simulink model "RCN_comparation"  (R2014b)
settings: Solver=ode45  StartTime=0.0  StopTime=4  RelTol=1e-3
libraries: NeuroModelerLibrary x31, simulink x4
settings Model: Creator=ai?  LastModifiedBy=Tim
settings DataIOCC: SignalLoggingSaveFormat=ModelDataLogs
settings OptimizationCC: ExpressionDepthLimit=2147483647
settings DebuggingCC: UnderspecifiedInitializationDetection=Classic  MergeDetectMultiDrivingBlocksExec=none  FcnCallInpInsideContextMsg=UseLocalSettings  StateNameClashWarn=warning
settings GRTTargetCC: CombineOutputUpdateFcns=off  GRTInterface=on

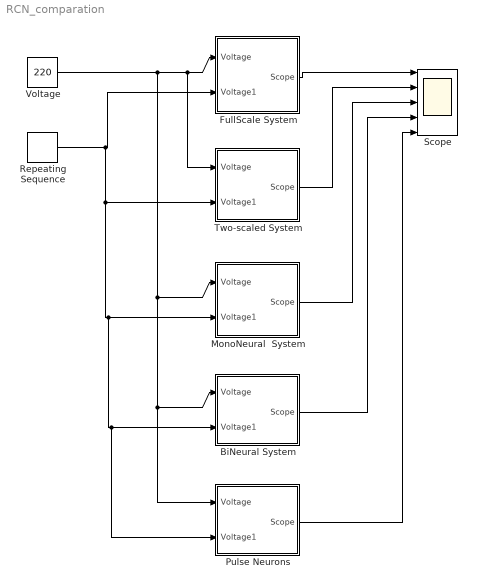
== system RCN_comparation ==
  BiNeural System : Subsystem
  FullScale System : Subsystem
  MonoNeural  System : Subsystem
  Pulse Neurons : Subsystem
  Repeating Sequence : simulink/Sources/Repeating Sequence  rep_seq_t=[0 1 1.01 2 2.01 3 3.01 4 4.01 10]  rep_seq_y=[3 3 1 1 -2 -2 -1 -1 20 20]
  Scope : Scope  NumInputPorts=5
      settings: YMin=0~0~0~0~-500  YMax=5~200~4~4~500  MaxDataPoints=500000
  Two-scaled System : Subsystem
  Voltage : Constant  Value=220
  wires:
  FullScale System/1(Scope) -> Scope/1
  Two-scaled System/1(Scope) -> Scope/2
  MonoNeural  System/1(Scope) -> Scope/3
  BiNeural System/1(Scope) -> Scope/4
  Pulse Neurons/1(Scope) -> Scope/5
  Voltage/1 -> FullScale System/1(Voltage), Two-scaled System/1(Voltage), MonoNeural  System/1(Voltage), BiNeural System/1(Voltage), Pulse Neurons/1(Voltage)
  Repeating Sequence/1 -> Pulse Neurons/2(Voltage1), BiNeural System/2(Voltage1), MonoNeural  System/2(Voltage1), Two-scaled System/2(Voltage1), FullScale System/2(Voltage1)

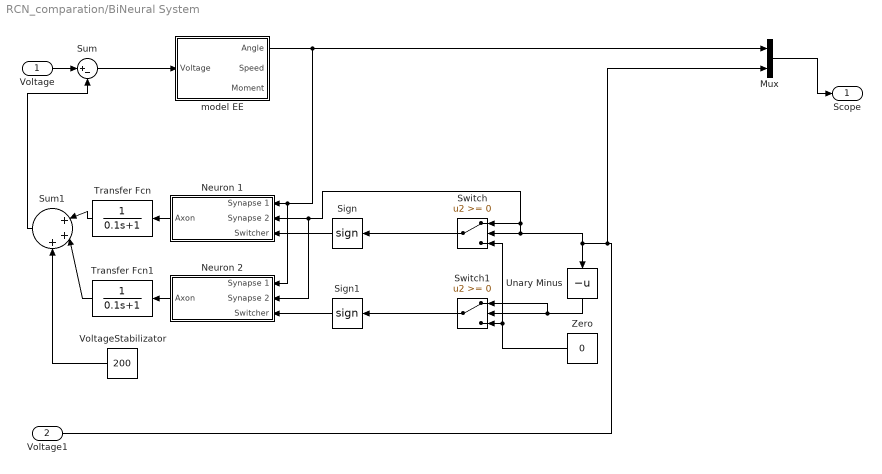
== system RCN_comparation/BiNeural System ==
  Voltage : Inport
  Voltage1 : Inport  Port=2
  Mux : Mux  Inputs=2
  Neuron 1 : Subsystem
  Neuron 2 : Subsystem
  Sign : Signum
  Sign1 : Signum
  Sum : Sum  Inputs=|+-
  Sum1 : Sum  Inputs=|+++
  Switch : Switch
  Switch1 : Switch
  Transfer Fcn : TransferFcn  Denominator=[0.1 1]
  Transfer Fcn1 : TransferFcn  Denominator=[0.1 1]
  Unary Minus : UnaryMinus
  VoltageStabilizator : Constant  Value=200
  Zero : Constant  Value=0
  model EE : Subsystem
  Scope : Outport
  wires:
  model EE/1(Angle) -> Mux/1, Neuron 1/1(Synapse 1), Neuron 2/1(Synapse 1)
  Voltage/1 -> Sum/1
  Mux/1 -> Scope/1
  Sum/1 -> model EE/1(Voltage)
  Neuron 1/1(Axon) -> Transfer Fcn/1
  Sum1/1 -> Sum/2
  Neuron 2/1(Axon) -> Transfer Fcn1/1
  Switch/1 -> Sign/1
  Switch1/1 -> Sign1/1
  Unary Minus/1 -> Switch1/2, Switch1/1
  Zero/1 -> Switch1/3, Switch/3
  Sign1/1 -> Neuron 2/3(Switcher)
  Sign/1 -> Neuron 1/3(Switcher)
  Transfer Fcn/1 -> Sum1/1
  Transfer Fcn1/1 -> Sum1/2
  VoltageStabilizator/1 -> Sum1/3
  Voltage1/1 -> Mux/2, Unary Minus/1, Neuron 2/2(Synapse 2), Neuron 1/2(Synapse 2), Switch/1, Switch/2

== system RCN_comparation/FullScale System ==
  Voltage : Inport
  Voltage1 : Inport  Port=2
  Angle Needed : Constant  Value=3
  Control Unit : Subsystem
  Manual Switch : ManualSwitch  CurrentSetting=0
  Mux : Mux  Inputs=2
  PID Controller : simulink/Continuous/PID Controller  Controller=PI  TimeDomain=Continuous-time  SampleTime=-1  IntegratorMethod=Forward Euler  FilterMethod=Forward Euler  Form=Parallel  P=1.41465294803961  I=22.6639520121412  D=0.242701786704104  N=12.4632340746272  InitialConditionSource=internal  InitialConditionForIntegrator=0  InitialConditionForFilter=0  ExternalReset=none  LimitOutput=off  UpperSaturationLimit=inf  LowerSaturationLimit=-inf  LinearizeAsGain=off  AntiWindupMode=none  Kb=1  TrackingMode=off  Kt=1  PParamMin=[]  PParamMax=[]  IParamMin=[]  IParamMax=[]  DParamMin=[]  DParamMax=[]  NParamMin=[]  NParamMax=[]  KbParamMin=[]  KbParamMax=[]  KtParamMin=[]  KtParamMax=[]  POutMin=[]  POutMax=[]  IOutMin=[]  IOutMax=[]  DOutMin=[]  DOutMax=[]  NOutMin=[]  NOutMax=[]  KbOutMin=[]  KbOutMax=[]  KtOutMin=[]  KtOutMax=[]  IntegratorOutMin=[]  IntegratorOutMax=[]  FilterOutMin=[]  FilterOutMax=[]  SumOutMin=[]  SumOutMax=[]  SumI1OutMin=[]  SumI1OutMax=[]  SumI2OutMin=[]  SumI2OutMax=[]  SumI3OutMin=[]  SumI3OutMax=[]  SumDOutMin=[]  SumDOutMax=[]  SaturationOutMin=[]  SaturationOutMax=[]  IntegratorContinuousStateAttributes=''  IntegratorStateMustResolveToSignalObject=off  IntegratorRTWStateStorageClass=Auto  FilterContinuousStateAttributes=''  FilterStateMustResolveToSignalObject=off  FilterRTWStateStorageClass=Auto  DifferentiatorICPrevScaledInput=0  DifferentiatorOutMin=[]  DifferentiatorOutMax=[]  UseFilter=on
  Sum : Sum  Inputs=|+-
  model EE : Subsystem
  Scope : Outport
  wires:
  model EE/1(Angle) -> Mux/1, Control Unit/1(In1)
  Voltage/1 -> Sum/1
  Angle Needed/1 -> Manual Switch/1
  Manual Switch/1 -> Control Unit/2(In2)
  Mux/1 -> Scope/1
  PID Controller/1 -> model EE/1(Voltage)
  Sum/1 -> PID Controller/1
  Control Unit/1(Out1) -> Sum/2
  Voltage1/1 -> Mux/2, Manual Switch/2

== system RCN_comparation/MonoNeural  System ==
  Voltage : Inport
  Voltage1 : Inport  Port=2
  Mux : Mux  Inputs=2
  Neuron 1 : Subsystem
  Sum : Sum  Inputs=|+-
  Sum1 : Sum  Inputs=|++
  Switcher : Constant
  Transfer Fcn : TransferFcn  Denominator=[0.01 1]
  VoltageStabilizator : Constant  Value=200
  model EE : Subsystem
  Scope : Outport
  wires:
  model EE/1(Angle) -> Mux/1, Neuron 1/1(Synapse 1)
  Voltage/1 -> Sum/1
  Mux/1 -> Scope/1
  Sum/1 -> model EE/1(Voltage)
  Neuron 1/1(Axon) -> Transfer Fcn/1
  Sum1/1 -> Sum/2
  Switcher/1 -> Neuron 1/3(Switcher)
  Transfer Fcn/1 -> Sum1/2
  VoltageStabilizator/1 -> Sum1/1
  Voltage1/1 -> Mux/2, Neuron 1/2(Synapse 2)

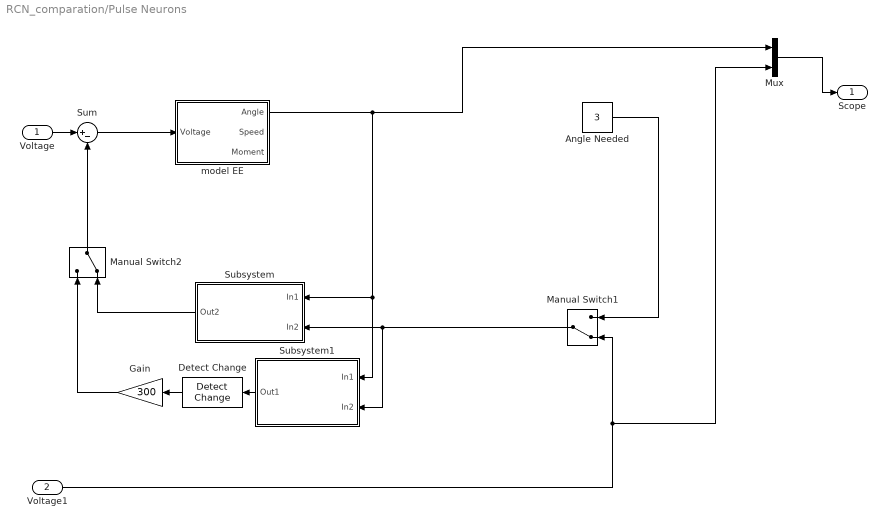
== system RCN_comparation/Pulse Neurons ==
  Voltage : Inport
  Voltage1 : Inport  Port=2
  Angle Needed : Constant  Value=3
  Detect Change : simulink/Logic and Bit Operations/Detect Change  vinit=0  InputProcessing=Inherited  OutDataTypeStr=uint8
  Gain : Gain  Gain=300
  Manual Switch1 : ManualSwitch  CurrentSetting=0
  Manual Switch2 : ManualSwitch  CurrentSetting=0
  Mux : Mux  Inputs=2
  Subsystem : Subsystem
  Subsystem1 : Subsystem
  Sum : Sum  Inputs=|+-
  model EE : Subsystem
  Scope : Outport
  wires:
  model EE/1(Angle) -> Mux/1, Subsystem/1(In1), Subsystem1/1(In1)
  Angle Needed/1 -> Manual Switch1/1
  Mux/1 -> Scope/1
  Sum/1 -> model EE/1(Voltage)
  Manual Switch1/1 -> Subsystem/2(In2), Subsystem1/2(In2)
  Voltage/1 -> Sum/1
  Subsystem/1(Out2) -> Manual Switch2/2
  Gain/1 -> Manual Switch2/1
  Detect Change/1 -> Gain/1
  Subsystem1/1(Out1) -> Detect Change/1
  Manual Switch2/1 -> Sum/2
  Voltage1/1 -> Manual Switch1/2, Mux/2

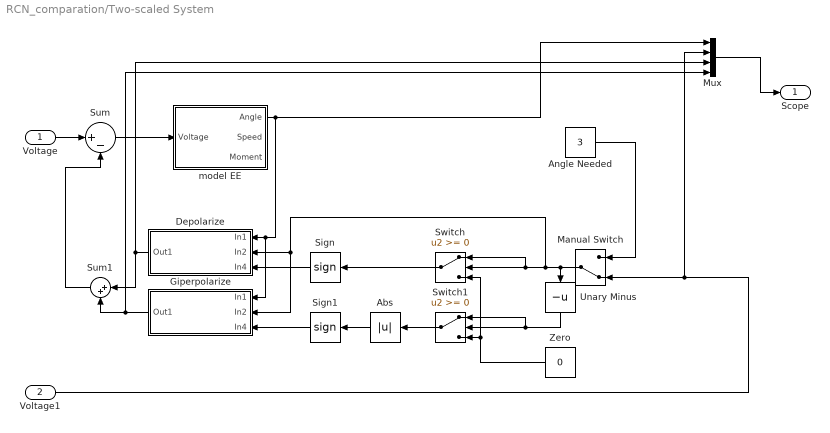
== system RCN_comparation/Two-scaled System ==
  Voltage : Inport
  Voltage1 : Inport  Port=2
  Abs : Abs
  Angle Needed : Constant  Value=3
  Depolarize : Subsystem
  Giperpolarize : Subsystem
  Manual Switch : ManualSwitch  CurrentSetting=0
  Mux : Mux
  Sign : Signum
  Sign1 : Signum
  Sum : Sum  Inputs=|+-
  Sum1 : Sum  Inputs=|++
  Switch : Switch
  Switch1 : Switch
  Unary Minus : UnaryMinus
  Zero : Constant  Value=0
  model EE : Subsystem
  Scope : Outport
  wires:
  model EE/1(Angle) -> Mux/1, Giperpolarize/1(In1), Depolarize/1(In1)
  Voltage/1 -> Sum/1
  Angle Needed/1 -> Manual Switch/1
  Mux/1 -> Scope/1
  Sum/1 -> model EE/1(Voltage)
  Manual Switch/1 -> Unary Minus/1, Switch/2, Switch/1, Depolarize/2(In2), Giperpolarize/2(In2)
  Sum1/1 -> Sum/2
  Depolarize/1(Out1) -> Sum1/1, Mux/3
  Giperpolarize/1(Out1) -> Sum1/2, Mux/4
  Switch/1 -> Sign/1
  Switch1/1 -> Abs/1
  Unary Minus/1 -> Switch1/2, Switch1/1
  Zero/1 -> Switch1/3, Switch/3
  Sign/1 -> Depolarize/3(In4)
  Abs/1 -> Sign1/1
  Sign1/1 -> Giperpolarize/3(In4)
  Voltage1/1 -> Mux/2, Manual Switch/2

== system RCN_comparation/BiNeural System/Neuron 1 ==
  Synapse 1 : Inport
  Synapse 2 : Inport  Port=2
  Switcher : Inport  Port=3
  Constant : Constant  Value=300
  Fcn : Fcn  Expr=tanh(u)
  Product : Product  Inputs=3  RndMeth=Zero
  Sum : Sum  Inputs=|++
  Weight 1 : Gain  Gain=5
  Weight 2 : Gain  Gain=-5
  Axon : Outport
  wires:
  Synapse 1/1 -> Weight 1/1
  Synapse 2/1 -> Weight 2/1
  Weight 1/1 -> Sum/1
  Weight 2/1 -> Sum/2
  Sum/1 -> Fcn/1
  Fcn/1 -> Product/1
  Product/1 -> Axon/1
  Constant/1 -> Product/2
  Switcher/1 -> Product/3

== system RCN_comparation/BiNeural System/Neuron 2 ==
  Synapse 1 : Inport
  Synapse 2 : Inport  Port=2
  Switcher : Inport  Port=3
  Constant : Constant  Value=300
  Fcn : Fcn  Expr=tanh(u)
  Product : Product  Inputs=3  RndMeth=Zero
  Sum : Sum  Inputs=|++
  Weight 1 : Gain  Gain=5
  Weight 2 : Gain  Gain=-5
  Axon : Outport
  wires:
  Switcher/1 -> Product/3
  Constant/1 -> Product/2
  Product/1 -> Axon/1
  Fcn/1 -> Product/1
  Sum/1 -> Fcn/1
  Weight 2/1 -> Sum/2
  Weight 1/1 -> Sum/1
  Synapse 2/1 -> Weight 2/1
  Synapse 1/1 -> Weight 1/1

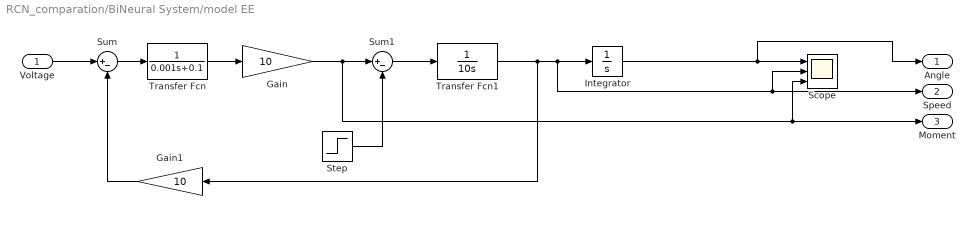
== system RCN_comparation/BiNeural System/model EE ==
  Voltage : Inport
  Gain : Gain  Gain=10
  Gain1 : Gain  Gain=10
  Integrator : Integrator
  Scope : Scope  NumInputPorts=3
      settings: YMin=-700000~-4.5e+008~-1.5e+006  YMax=100000~5e+007~250000
  Step : Step  Time=0.2  After=2500  SampleTime=0
  Sum : Sum  Inputs=|+-
  Sum1 : Sum  Inputs=|+-
  Transfer Fcn : TransferFcn  Denominator=[0.001 0.1]
  Transfer Fcn1 : TransferFcn  Denominator=[10 0]
  Angle : Outport  Tag=Angle
  Speed : Outport  Port=2
  Moment : Outport  Port=3
  wires:
  Voltage/1 -> Sum/1
  Sum/1 -> Transfer Fcn/1
  Transfer Fcn/1 -> Gain/1
  Sum1/1 -> Transfer Fcn1/1
  Transfer Fcn1/1 -> Integrator/1, Scope/2, Speed/1, Gain1/1
  Gain1/1 -> Sum/2
  Step/1 -> Sum1/2
  Integrator/1 -> Angle/1, Scope/1
  Gain/1 -> Sum1/1, Moment/1, Scope/3

== system RCN_comparation/FullScale System/Control Unit ==
  In1 : Inport
  In2 : Inport  Port=2
  Abs : Abs
  Constant : Constant  Value=220
  Divide : Product  Inputs=*/
  In3 : InportShadow  Port=2
  Product : Product  RndMeth=Zero
  Sum : Sum  Inputs=|+-
  Sum1 : Sum  Inputs=|++
  Out1 : Outport
  wires:
  In1/1 -> Sum/1
  In2/1 -> Sum/2
  Constant/1 -> Divide/1, Sum1/1
  In3/1 -> Abs/1
  Divide/1 -> Product/1
  Sum/1 -> Product/2
  Product/1 -> Sum1/2
  Sum1/1 -> Out1/1
  Abs/1 -> Divide/2

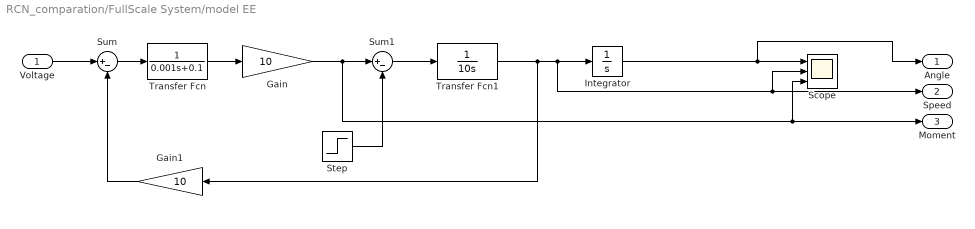
== system RCN_comparation/FullScale System/model EE ==
  Voltage : Inport
  Gain : Gain  Gain=10
  Gain1 : Gain  Gain=10
  Integrator : Integrator
  Scope : Scope  NumInputPorts=3
      settings: YMin=-700000~-4.5e+008~-1.5e+006  YMax=100000~5e+007~250000
  Step : Step  Time=0.2  After=2500  SampleTime=0
  Sum : Sum  Inputs=|+-
  Sum1 : Sum  Inputs=|+-
  Transfer Fcn : TransferFcn  Denominator=[0.001 0.1]
  Transfer Fcn1 : TransferFcn  Denominator=[10 0]
  Angle : Outport  Tag=Angle
  Speed : Outport  Port=2
  Moment : Outport  Port=3
  wires:
  Voltage/1 -> Sum/1
  Sum/1 -> Transfer Fcn/1
  Transfer Fcn/1 -> Gain/1
  Sum1/1 -> Transfer Fcn1/1
  Transfer Fcn1/1 -> Integrator/1, Scope/2, Speed/1, Gain1/1
  Gain1/1 -> Sum/2
  Step/1 -> Sum1/2
  Integrator/1 -> Angle/1, Scope/1
  Gain/1 -> Sum1/1, Moment/1, Scope/3

== system RCN_comparation/MonoNeural  System/Neuron 1 ==
  Synapse 1 : Inport
  Synapse 2 : Inport  Port=2
  Switcher : Inport  Port=3
  Constant : Constant  Value=300
  Fcn : Fcn  Expr=tanh(u)
  Product : Product  Inputs=3  RndMeth=Zero
  Sum : Sum  Inputs=|++
  Weight 1 : Gain  Gain=5
  Weight 2 : Gain  Gain=-5
  Axon : Outport
  wires:
  Synapse 1/1 -> Weight 1/1
  Synapse 2/1 -> Weight 2/1
  Weight 1/1 -> Sum/1
  Weight 2/1 -> Sum/2
  Sum/1 -> Fcn/1
  Fcn/1 -> Product/1
  Product/1 -> Axon/1
  Constant/1 -> Product/2
  Switcher/1 -> Product/3

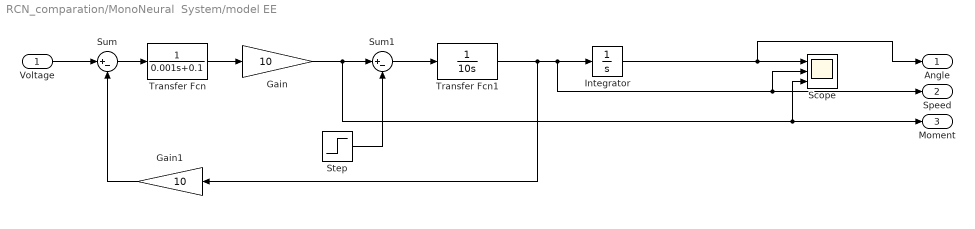
== system RCN_comparation/MonoNeural  System/model EE ==
  Voltage : Inport
  Gain : Gain  Gain=10
  Gain1 : Gain  Gain=10
  Integrator : Integrator
  Scope : Scope  NumInputPorts=3
      settings: YMin=-700000~-4.5e+008~-1.5e+006  YMax=100000~5e+007~250000
  Step : Step  Time=0.2  After=2500  SampleTime=0
  Sum : Sum  Inputs=|+-
  Sum1 : Sum  Inputs=|+-
  Transfer Fcn : TransferFcn  Denominator=[0.001 0.1]
  Transfer Fcn1 : TransferFcn  Denominator=[10 0]
  Angle : Outport  Tag=Angle
  Speed : Outport  Port=2
  Moment : Outport  Port=3
  wires:
  Voltage/1 -> Sum/1
  Sum/1 -> Transfer Fcn/1
  Transfer Fcn/1 -> Gain/1
  Sum1/1 -> Transfer Fcn1/1
  Transfer Fcn1/1 -> Integrator/1, Scope/2, Speed/1, Gain1/1
  Gain1/1 -> Sum/2
  Step/1 -> Sum1/2
  Integrator/1 -> Angle/1, Scope/1
  Gain/1 -> Sum1/1, Moment/1, Scope/3

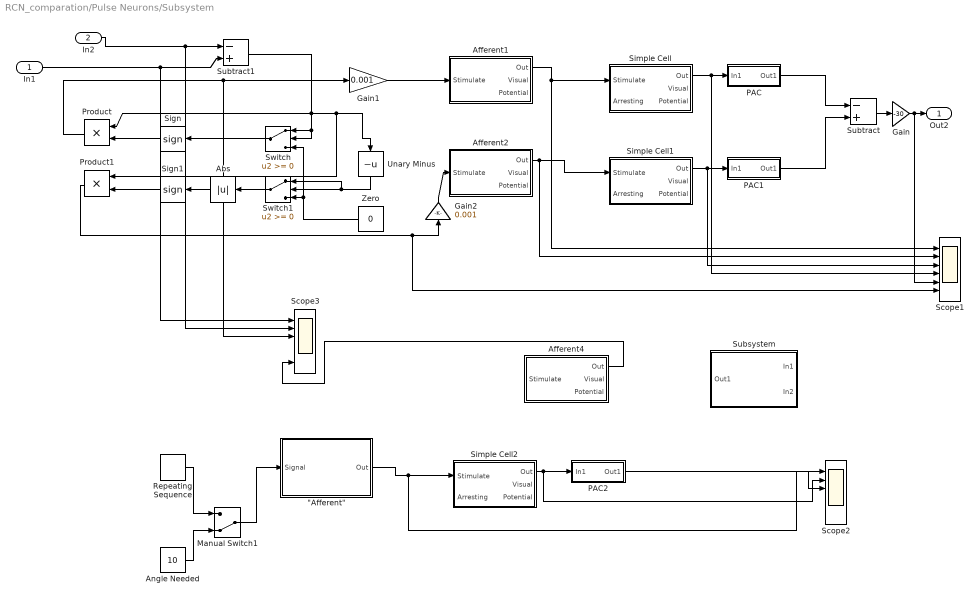
== system RCN_comparation/Pulse Neurons/Subsystem ==
  In1 : Inport
  In2 : Inport  Port=2
  "\"Afferent\"" : Subsystem
  Abs : Abs
  Afferent1 : Subsystem  AncestorBlock=NeuroModelerLibrary/Simple Cells/Afferent1
  Afferent2 : Subsystem  AncestorBlock=NeuroModelerLibrary/Simple Cells/Afferent1
  Afferent4 : Subsystem  AncestorBlock=NeuroModelerLibrary/Simple Cells/Afferent1
  Angle Needed : Constant  Value=10
  Gain : Gain  Gain=-30
  Gain1 : Gain  Gain=0.001
  Gain2 : Gain  Gain=0.001
  Manual Switch1 : ManualSwitch  CurrentSetting=0
  PAC : Subsystem  AncestorBlock=NeuroModelerLibrary/Neuron Elements/Synapse  mask{SecretionTC=0.001, DecompositionTC=0.1, ksi=2, gamma=1e8}
      mask prompts: SecretionTC "Mediator Secretion"; DecompositionTC "Mediator Decomposition"
  PAC1 : Subsystem  AncestorBlock=NeuroModelerLibrary/Neuron Elements/Synapse  mask{SecretionTC=0.001, DecompositionTC=0.1, ksi=2, gamma=1e8}
      mask prompts: SecretionTC "Mediator Secretion"; DecompositionTC "Mediator Decomposition"
  PAC2 : Subsystem  AncestorBlock=NeuroModelerLibrary/Neuron Elements/Synapse  mask{SecretionTC=0.001, DecompositionTC=0.1, ksi=2, gamma=1e8}
      mask prompts: SecretionTC "Mediator Secretion"; DecompositionTC "Mediator Decomposition"
  Product : Product  RndMeth=Zero
  Product1 : Product  RndMeth=Zero
  Repeating Sequence : simulink/Sources/Repeating Sequence  rep_seq_t=[0 1 1.01 2 2.01 3 3.01 4 4.01 10]  rep_seq_y=[3 3 1 1 -2 -2 -1 -1 20 20]
  Scope1 : Scope  NumInputPorts=6
      settings: TickLabels=on  TimeRange=4  YMin=0~-1~-1~0~2700~-500  YMax=1~1~1~1~2900~0  SaveName=ScopeData2  MaxDataPoints=500000
  Scope2 : Scope  NumInputPorts=6
      settings: TickLabels=on  TimeRange=4  YMin=-1~-1~-1~-1~-1~0.65  YMax=1~1~1~1~1~1  SaveName=ScopeData3  MaxDataPoints=500000
  Scope3 : Scope  NumInputPorts=6
      settings: TickLabels=on  TimeRange=4  YMin=1~3~-0~0~-0.7~-0  YMax=4.5~3~1.5~1~0.2~0.2  SaveName=ScopeData5  MaxDataPoints=500000
  Sign : Signum
  Sign1 : Signum
  Simple Cell : Subsystem  AncestorBlock=NeuroModelerLibrary/Simple Cells/Simple Cell
  Simple Cell1 : Subsystem  AncestorBlock=NeuroModelerLibrary/Simple Cells/Simple Cell
  Simple Cell2 : Subsystem  AncestorBlock=NeuroModelerLibrary/Simple Cells/Simple Cell
  Subsystem : Subsystem
  Subtract : Sum  Inputs=-+
  Subtract1 : Sum  Inputs=-+
  Switch : Switch
  Switch1 : Switch
  Unary Minus : UnaryMinus
  Zero : Constant  Value=0
  Out2 : Outport
  wires:
  Afferent1/1(Out) -> Scope1/1, Simple Cell/1(Stimulate)
  Simple Cell1/1(Out) -> PAC1/1(In1), Scope1/3
  Afferent2/1(Out) -> Scope1/2, Simple Cell1/1(Stimulate)
  Simple Cell/1(Out) -> PAC/1(In1), Scope1/4
  PAC/1(Out1) -> Subtract/1
  PAC1/1(Out1) -> Subtract/2
  Subtract/1 -> Gain/1
  Gain/1 -> Out2/1, Scope1/5
  Switch/1 -> Sign/1
  Switch1/1 -> Abs/1
  Unary Minus/1 -> Switch1/2, Switch1/1
  Zero/1 -> Switch1/3, Switch/3
  Sign/1 -> Product/2
  Abs/1 -> Sign1/1
  Sign1/1 -> Product1/2
  Product/1 -> Scope3/3, Gain1/1
  Product1/1 -> Gain2/1, Scope1/6
  Subtract1/1 -> Switch/2, Switch/1, Product/1, Unary Minus/1, Product1/1
  Gain1/1 -> Afferent1/1(Stimulate)
  Gain2/1 -> Afferent2/1(Stimulate)
  Afferent4/1(Out) -> Scope3/6
  "\"Afferent\""/1(Out) -> Simple Cell2/1(Stimulate), Scope2/1
  Simple Cell2/1(Out) -> PAC2/1(In1), Scope2/2
  In2/1 -> Subtract1/1, Scope3/2
  In1/1 -> Subtract1/2, Scope3/1
  PAC2/1(Out1) -> Scope2/3
  Manual Switch1/1 -> "\"Afferent\""/1(Signal)
  Repeating Sequence/1 -> Manual Switch1/1
  Angle Needed/1 -> Manual Switch1/2

== system RCN_comparation/Pulse Neurons/Subsystem1 ==
  In1 : Inport
  In2 : Inport  Port=2
  "\"Afferent\"1" : Subsystem
  PAC3 : Subsystem  AncestorBlock=NeuroModelerLibrary/Neuron Elements/Synapse  mask{SecretionTC=0.001, DecompositionTC=0.1, ksi=2, gamma=1e8}
      mask prompts: SecretionTC "Mediator Secretion"; DecompositionTC "Mediator Decomposition"
  Simple Cell3 : Subsystem  AncestorBlock=NeuroModelerLibrary/Simple Cells/Simple Cell
  Subtract2 : Sum  Inputs=-+
  Out1 : Outport
  wires:
  "\"Afferent\"1"/1(Out) -> Simple Cell3/1(Stimulate)
  Simple Cell3/1(Out) -> PAC3/1(In1)
  Subtract2/1 -> "\"Afferent\"1"/1(Signal)
  In1/1 -> Subtract2/1
  PAC3/1(Out1) -> Out1/1
  In2/1 -> Subtract2/2

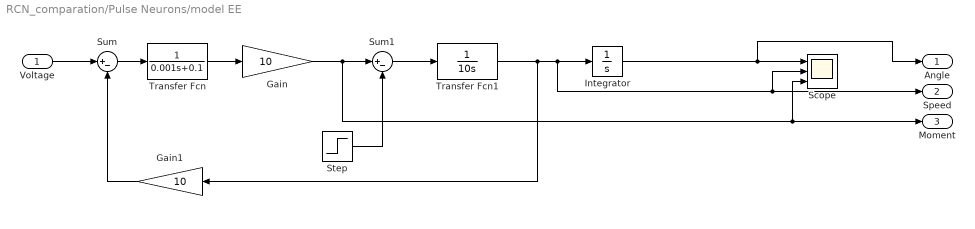
== system RCN_comparation/Pulse Neurons/model EE ==
  Voltage : Inport
  Gain : Gain  Gain=10
  Gain1 : Gain  Gain=10
  Integrator : Integrator
  Scope : Scope  NumInputPorts=3
      settings: YMin=-700000~-4.5e+008~-1.5e+006  YMax=100000~5e+007~250000
  Step : Step  Time=0.2  After=2500  SampleTime=0
  Sum : Sum  Inputs=|+-
  Sum1 : Sum  Inputs=|+-
  Transfer Fcn : TransferFcn  Denominator=[0.001 0.1]
  Transfer Fcn1 : TransferFcn  Denominator=[10 0]
  Angle : Outport  Tag=Angle
  Speed : Outport  Port=2
  Moment : Outport  Port=3
  wires:
  Voltage/1 -> Sum/1
  Sum/1 -> Transfer Fcn/1
  Transfer Fcn/1 -> Gain/1
  Sum1/1 -> Transfer Fcn1/1
  Transfer Fcn1/1 -> Integrator/1, Scope/2, Speed/1, Gain1/1
  Gain1/1 -> Sum/2
  Step/1 -> Sum1/2
  Integrator/1 -> Angle/1, Scope/1
  Gain/1 -> Sum1/1, Moment/1, Scope/3

== system RCN_comparation/Two-scaled System/Depolarize ==
  In1 : Inport
  In2 : Inport  Port=2
  In4 : Inport  Port=3
  Abs : Abs
  Constant : Constant  Value=220
  Divide : Product  Inputs=*/
  In3 : InportShadow  Port=2
  Product : Product  RndMeth=Zero
  Product1 : Product  RndMeth=Zero
  Sum : Sum  Inputs=|+-
  Sum1 : Sum  Inputs=|++
  Out1 : Outport
  wires:
  In1/1 -> Sum/1
  In2/1 -> Sum/2
  Constant/1 -> Divide/1, Sum1/1
  In3/1 -> Abs/1
  Divide/1 -> Product/1
  Sum/1 -> Product/2
  Product/1 -> Sum1/2
  Sum1/1 -> Product1/1
  Product1/1 -> Out1/1
  In4/1 -> Product1/2
  Abs/1 -> Divide/2

== system RCN_comparation/Two-scaled System/Giperpolarize ==
  In1 : Inport
  In2 : Inport  Port=2
  In4 : Inport  Port=3
  Abs : Abs
  Constant : Constant  Value=220
  Divide : Product  Inputs=*/
  In3 : InportShadow  Port=2
  Product : Product  RndMeth=Zero
  Product1 : Product  RndMeth=Zero
  Sum : Sum  Inputs=|+-
  Sum1 : Sum  Inputs=|++
  Out1 : Outport
  wires:
  In4/1 -> Product1/2
  Product1/1 -> Out1/1
  Sum1/1 -> Product1/1
  Product/1 -> Sum1/2
  Sum/1 -> Product/2
  Divide/1 -> Product/1
  In3/1 -> Abs/1
  Constant/1 -> Sum1/1, Divide/1
  In2/1 -> Sum/2
  In1/1 -> Sum/1
  Abs/1 -> Divide/2

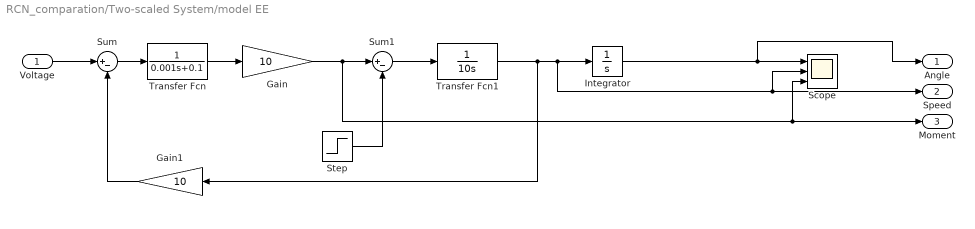
== system RCN_comparation/Two-scaled System/model EE ==
  Voltage : Inport
  Gain : Gain  Gain=10
  Gain1 : Gain  Gain=10
  Integrator : Integrator
  Scope : Scope  NumInputPorts=3
      settings: YMin=-700000~-4.5e+008~-1.5e+006  YMax=100000~5e+007~250000
  Step : Step  Time=0.2  After=2500  SampleTime=0
  Sum : Sum  Inputs=|+-
  Sum1 : Sum  Inputs=|+-
  Transfer Fcn : TransferFcn  Denominator=[0.001 0.1]
  Transfer Fcn1 : TransferFcn  Denominator=[10 0]
  Angle : Outport  Tag=Angle
  Speed : Outport  Port=2
  Moment : Outport  Port=3
  wires:
  Voltage/1 -> Sum/1
  Sum/1 -> Transfer Fcn/1
  Transfer Fcn/1 -> Gain/1
  Sum1/1 -> Transfer Fcn1/1
  Transfer Fcn1/1 -> Integrator/1, Scope/2, Speed/1, Gain1/1
  Gain1/1 -> Sum/2
  Step/1 -> Sum1/2
  Integrator/1 -> Angle/1, Scope/1
  Gain/1 -> Sum1/1, Moment/1, Scope/3

== system RCN_comparation/Pulse Neurons/Subsystem/"Afferent" ==
  Signal : Inport
  Clock : Clock
  Fcn : Fcn  Expr=sin(u)
  Product2 : Product  RndMeth=Zero
  Relay : Relay  OnSwitchValue=0.9  OffSwitchValue=0.9
  Out : Outport
  wires:
  Clock/1 -> Product2/1
  Product2/1 -> Fcn/1
  Signal/1 -> Product2/2
  Fcn/1 -> Relay/1
  Relay/1 -> Out/1

== system RCN_comparation/Pulse Neurons/Subsystem/Afferent1 ==
  Stimulate : Inport
  C1 : Constant
  C2 : Constant  Value=0
  C3 : Constant  Value=-1
  Fcn : Fcn  Expr=2-exp(-0.001*(u+0.99))
  LTZone : NeuroModelerLibrary/Neuron Elements/LTZone  NM=1  FB=0.08  IT=0.005  T=0.000001
  Simple Membrane1 : NeuroModelerLibrary/Neuron Elements/Simple Membrane  ACm=1e-7  ARm=1e7  ECm=1e-7  ERm=1e7  ARFm=1e8  ERFm=1e8
  Sum1 : Sum  SaturateOnIntegerOverflow=on  InputSameDT=on  OutDataTypeStr=Inherit: Same as first input
  Sum7 : Sum  SaturateOnIntegerOverflow=on  InputSameDT=on  OutDataTypeStr=Inherit: Same as first input
  Out : Outport
  Visual : Outport  Port=2
  Potential : Outport  Port=3
  wires:
  C3/1 -> Simple Membrane1/4
  Sum7/1 -> LTZone/1, Potential/1
  C1/1 -> LTZone/2
  LTZone/3 -> Out/1
  LTZone/2 -> Visual/1
  Simple Membrane1/1 -> Sum7/1
  Simple Membrane1/2 -> Sum7/2
  LTZone/1 -> Simple Membrane1/3
  C2/1 -> Sum1/2
  Stimulate/1 -> Fcn/1
  Sum1/1 -> Simple Membrane1/2
  Fcn/1 -> Sum1/1

== system RCN_comparation/Pulse Neurons/Subsystem/Afferent2 ==
  Stimulate : Inport
  C1 : Constant
  C2 : Constant  Value=-2
  C3 : Constant
  Fcn : Fcn  Expr=2-exp(-0.001*(u+0.99))
  LTZone : NeuroModelerLibrary/Neuron Elements/LTZone  NM=1  FB=0.08  IT=0.005  T=0.00001
  Simple Membrane1 : NeuroModelerLibrary/Neuron Elements/Simple Membrane  ACm=1e-9  ARm=1e7  ECm=1e-7  ERm=1e7  ARFm=1e8  ERFm=1e8
  Sum1 : Sum  SaturateOnIntegerOverflow=on  InputSameDT=on  OutDataTypeStr=Inherit: Same as first input
  Sum7 : Sum  SaturateOnIntegerOverflow=on  InputSameDT=on  OutDataTypeStr=Inherit: Same as first input
  Out : Outport
  Visual : Outport  Port=2
  Potential : Outport  Port=3
  wires:
  Sum7/1 -> LTZone/1, Potential/1
  C1/1 -> LTZone/2
  LTZone/3 -> Out/1
  LTZone/2 -> Visual/1
  Simple Membrane1/1 -> Sum7/1
  Simple Membrane1/2 -> Sum7/2
  LTZone/1 -> Simple Membrane1/3
  C2/1 -> Sum1/2
  Stimulate/1 -> Fcn/1
  Fcn/1 -> Sum1/1
  Sum1/1 -> Simple Membrane1/4
  C3/1 -> Simple Membrane1/2

== system RCN_comparation/Pulse Neurons/Subsystem/Afferent4 ==
  Stimulate : Inport
  C1 : Constant
  C2 : Constant  Value=0
  C3 : Constant  Value=-1
  Fcn : Fcn  Expr=2-exp(-0.001*u)
  LTZone : NeuroModelerLibrary/Neuron Elements/LTZone  NM=1  FB=0.08  IT=0.005  T=0.000001
  Simple Membrane1 : NeuroModelerLibrary/Neuron Elements/Simple Membrane  ACm=1e-7  ARm=1e7  ECm=1e-7  ERm=1e7  ARFm=1e8  ERFm=1e8
  Sum1 : Sum  SaturateOnIntegerOverflow=on  InputSameDT=on  OutDataTypeStr=Inherit: Same as first input
  Sum7 : Sum  SaturateOnIntegerOverflow=on  InputSameDT=on  OutDataTypeStr=Inherit: Same as first input
  Out : Outport
  Visual : Outport  Port=2
  Potential : Outport  Port=3
  wires:
  Fcn/1 -> Sum1/1
  Sum1/1 -> Simple Membrane1/2
  Stimulate/1 -> Fcn/1
  C2/1 -> Sum1/2
  LTZone/1 -> Simple Membrane1/3
  Simple Membrane1/2 -> Sum7/2
  Simple Membrane1/1 -> Sum7/1
  LTZone/2 -> Visual/1
  LTZone/3 -> Out/1
  C1/1 -> LTZone/2
  Sum7/1 -> Potential/1, LTZone/1
  C3/1 -> Simple Membrane1/4

== system RCN_comparation/Pulse Neurons/Subsystem/PAC ==
  In1 : Inport
  Constant4 : Constant  Value=DecompositionTC
  Constant5 : Constant  Value=SecretionTC
  Gain1 : Gain  SaturateOnIntegerOverflow=on  OutDataTypeStr=Inherit: Same as input  ParamDataTypeStr=Inherit: Same as input
  Inertial Link : NeuroModelerLibrary/Support/Inertial Link
  Switch2 : Switch  Threshold=1
  Out1 : Outport
  wires:
  In1/1 -> Switch2/2, Gain1/1
  Constant4/1 -> Switch2/3
  Constant5/1 -> Switch2/1
  Switch2/1 -> Inertial Link/2
  Gain1/1 -> Inertial Link/1
  Inertial Link/1 -> Out1/1

== system RCN_comparation/Pulse Neurons/Subsystem/PAC1 ==
  In1 : Inport
  Constant4 : Constant  Value=DecompositionTC
  Constant5 : Constant  Value=SecretionTC
  Gain1 : Gain  SaturateOnIntegerOverflow=on  OutDataTypeStr=Inherit: Same as input  ParamDataTypeStr=Inherit: Same as input
  Inertial Link : NeuroModelerLibrary/Support/Inertial Link
  Switch2 : Switch  Threshold=1
  Out1 : Outport
  wires:
  In1/1 -> Switch2/2, Gain1/1
  Constant4/1 -> Switch2/3
  Constant5/1 -> Switch2/1
  Switch2/1 -> Inertial Link/2
  Gain1/1 -> Inertial Link/1
  Inertial Link/1 -> Out1/1

== system RCN_comparation/Pulse Neurons/Subsystem/PAC2 ==
  In1 : Inport
  Constant4 : Constant  Value=DecompositionTC
  Constant5 : Constant  Value=SecretionTC
  Gain1 : Gain  SaturateOnIntegerOverflow=on  OutDataTypeStr=Inherit: Same as input  ParamDataTypeStr=Inherit: Same as input
  Inertial Link : NeuroModelerLibrary/Support/Inertial Link
  Switch2 : Switch  Threshold=1
  Out1 : Outport
  wires:
  In1/1 -> Switch2/2, Gain1/1
  Constant4/1 -> Switch2/3
  Constant5/1 -> Switch2/1
  Switch2/1 -> Inertial Link/2
  Gain1/1 -> Inertial Link/1
  Inertial Link/1 -> Out1/1

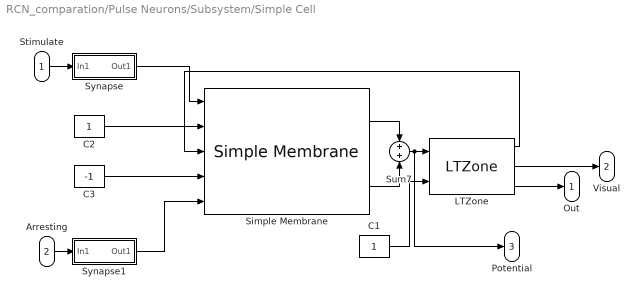
== system RCN_comparation/Pulse Neurons/Subsystem/Simple Cell ==
  Stimulate : Inport
  Arresting : Inport  Port=2
  C1 : Constant
  C2 : Constant
  C3 : Constant  Value=-1
  LTZone : NeuroModelerLibrary/Neuron Elements/LTZone  NM=1  FB=1.7  IT=0.005  T=0.000001
  Simple Membrane : NeuroModelerLibrary/Neuron Elements/Simple Membrane  ACm=1e-9  ARm=1e7  ECm=1e-9  ERm=1e7  ARFm=1e8  ERFm=1e8
  Sum7 : Sum  SaturateOnIntegerOverflow=on  InputSameDT=on  OutDataTypeStr=Inherit: Same as first input
  Synapse : Subsystem  AncestorBlock=NeuroModelerLibrary/Neuron Elements/Synapse  mask{SecretionTC=0.001, DecompositionTC=0.01, ksi=0.5, gamma=1e8}
      mask prompts: SecretionTC "Mediator Secretion"; DecompositionTC "Mediator Decomposition"
  Synapse1 : Subsystem  AncestorBlock=NeuroModelerLibrary/Neuron Elements/Synapse  mask{SecretionTC=0.001, DecompositionTC=0.01, ksi=0.5, gamma=1e8}
      mask prompts: SecretionTC "Mediator Secretion"; DecompositionTC "Mediator Decomposition"
  Out : Outport
  Visual : Outport  Port=2
  Potential : Outport  Port=3
  wires:
  Synapse1/1(Out1) -> Simple Membrane/5
  Synapse/1(Out1) -> Simple Membrane/1
  Simple Membrane/2 -> Sum7/2
  Simple Membrane/1 -> Sum7/1
  C3/1 -> Simple Membrane/4
  C2/1 -> Simple Membrane/2
  LTZone/1 -> Simple Membrane/3
  Sum7/1 -> Potential/1, LTZone/1
  Arresting/1 -> Synapse1/1(In1)
  Stimulate/1 -> Synapse/1(In1)
  C1/1 -> LTZone/2
  LTZone/3 -> Out/1
  LTZone/2 -> Visual/1

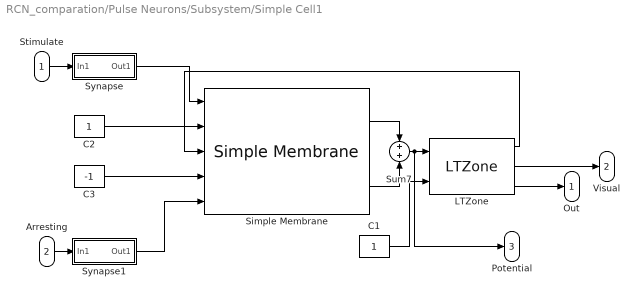
== system RCN_comparation/Pulse Neurons/Subsystem/Simple Cell1 ==
  Stimulate : Inport
  Arresting : Inport  Port=2
  C1 : Constant
  C2 : Constant
  C3 : Constant  Value=-1
  LTZone : NeuroModelerLibrary/Neuron Elements/LTZone  NM=1  FB=1.7  IT=0.005  T=0.000001
  Simple Membrane : NeuroModelerLibrary/Neuron Elements/Simple Membrane  ACm=1e-9  ARm=1e7  ECm=1e-9  ERm=1e7  ARFm=1e8  ERFm=1e8
  Sum7 : Sum  SaturateOnIntegerOverflow=on  InputSameDT=on  OutDataTypeStr=Inherit: Same as first input
  Synapse : Subsystem  AncestorBlock=NeuroModelerLibrary/Neuron Elements/Synapse  mask{SecretionTC=0.001, DecompositionTC=0.01, ksi=0.5, gamma=1e8}
      mask prompts: SecretionTC "Mediator Secretion"; DecompositionTC "Mediator Decomposition"
  Synapse1 : Subsystem  AncestorBlock=NeuroModelerLibrary/Neuron Elements/Synapse  mask{SecretionTC=0.001, DecompositionTC=0.01, ksi=0.5, gamma=1e8}
      mask prompts: SecretionTC "Mediator Secretion"; DecompositionTC "Mediator Decomposition"
  Out : Outport
  Visual : Outport  Port=2
  Potential : Outport  Port=3
  wires:
  Synapse1/1(Out1) -> Simple Membrane/5
  Synapse/1(Out1) -> Simple Membrane/1
  Simple Membrane/2 -> Sum7/2
  Simple Membrane/1 -> Sum7/1
  C3/1 -> Simple Membrane/4
  C2/1 -> Simple Membrane/2
  LTZone/1 -> Simple Membrane/3
  Sum7/1 -> Potential/1, LTZone/1
  Arresting/1 -> Synapse1/1(In1)
  Stimulate/1 -> Synapse/1(In1)
  C1/1 -> LTZone/2
  LTZone/3 -> Out/1
  LTZone/2 -> Visual/1

== system RCN_comparation/Pulse Neurons/Subsystem/Simple Cell2 ==
  Stimulate : Inport
  Arresting : Inport  Port=2
  C1 : Constant
  C2 : Constant
  C3 : Constant  Value=-1
  LTZone : NeuroModelerLibrary/Neuron Elements/LTZone  NM=1  FB=1.7  IT=0.005  T=0.000001
  Simple Membrane : NeuroModelerLibrary/Neuron Elements/Simple Membrane  ACm=1e-9  ARm=1e7  ECm=1e-9  ERm=1e7  ARFm=1e8  ERFm=1e8
  Sum7 : Sum  SaturateOnIntegerOverflow=on  InputSameDT=on  OutDataTypeStr=Inherit: Same as first input
  Synapse : Subsystem  AncestorBlock=NeuroModelerLibrary/Neuron Elements/Synapse  mask{SecretionTC=0.001, DecompositionTC=0.01, ksi=0.5, gamma=1e8}
      mask prompts: SecretionTC "Mediator Secretion"; DecompositionTC "Mediator Decomposition"
  Synapse1 : Subsystem  AncestorBlock=NeuroModelerLibrary/Neuron Elements/Synapse  mask{SecretionTC=0.001, DecompositionTC=0.01, ksi=0.5, gamma=1e8}
      mask prompts: SecretionTC "Mediator Secretion"; DecompositionTC "Mediator Decomposition"
  Out : Outport
  Visual : Outport  Port=2
  Potential : Outport  Port=3
  wires:
  Synapse1/1(Out1) -> Simple Membrane/5
  Synapse/1(Out1) -> Simple Membrane/1
  Simple Membrane/2 -> Sum7/2
  Simple Membrane/1 -> Sum7/1
  C3/1 -> Simple Membrane/4
  C2/1 -> Simple Membrane/2
  LTZone/1 -> Simple Membrane/3
  Sum7/1 -> Potential/1, LTZone/1
  Arresting/1 -> Synapse1/1(In1)
  Stimulate/1 -> Synapse/1(In1)
  C1/1 -> LTZone/2
  LTZone/3 -> Out/1
  LTZone/2 -> Visual/1

== system RCN_comparation/Pulse Neurons/Subsystem/Subsystem ==
  In1 : Inport
  In2 : Inport  Port=2
  "\"Afferent\"1" : Subsystem
  PAC3 : Subsystem  AncestorBlock=NeuroModelerLibrary/Neuron Elements/Synapse  mask{SecretionTC=0.001, DecompositionTC=0.1, ksi=2, gamma=1e8}
      mask prompts: SecretionTC "Mediator Secretion"; DecompositionTC "Mediator Decomposition"
  Simple Cell3 : Subsystem  AncestorBlock=NeuroModelerLibrary/Simple Cells/Simple Cell
  Subtract2 : Sum  Inputs=-+
  Out1 : Outport
  wires:
  "\"Afferent\"1"/1(Out) -> Simple Cell3/1(Stimulate)
  Simple Cell3/1(Out) -> PAC3/1(In1)
  Subtract2/1 -> "\"Afferent\"1"/1(Signal)
  In1/1 -> Subtract2/1
  PAC3/1(Out1) -> Out1/1
  In2/1 -> Subtract2/2

== system RCN_comparation/Pulse Neurons/Subsystem1/"Afferent"1 ==
  Signal : Inport
  Clock : Clock
  Fcn : Fcn  Expr=sin(u)
  Product2 : Product  RndMeth=Zero
  Relay : Relay  OnSwitchValue=0.9  OffSwitchValue=0.9
  Out : Outport
  wires:
  Clock/1 -> Product2/1
  Product2/1 -> Fcn/1
  Signal/1 -> Product2/2
  Fcn/1 -> Relay/1
  Relay/1 -> Out/1

== system RCN_comparation/Pulse Neurons/Subsystem1/PAC3 ==
  In1 : Inport
  Constant4 : Constant  Value=DecompositionTC
  Constant5 : Constant  Value=SecretionTC
  Gain1 : Gain  SaturateOnIntegerOverflow=on  OutDataTypeStr=Inherit: Same as input  ParamDataTypeStr=Inherit: Same as input
  Inertial Link : NeuroModelerLibrary/Support/Inertial Link
  Switch2 : Switch  Threshold=1
  Out1 : Outport
  wires:
  In1/1 -> Switch2/2, Gain1/1
  Constant4/1 -> Switch2/3
  Constant5/1 -> Switch2/1
  Switch2/1 -> Inertial Link/2
  Gain1/1 -> Inertial Link/1
  Inertial Link/1 -> Out1/1

== system RCN_comparation/Pulse Neurons/Subsystem1/Simple Cell3 ==
  Stimulate : Inport
  Arresting : Inport  Port=2
  C1 : Constant
  C2 : Constant
  C3 : Constant  Value=-1
  LTZone : NeuroModelerLibrary/Neuron Elements/LTZone  NM=1  FB=1.7  IT=0.005  T=0.000001
  Simple Membrane : NeuroModelerLibrary/Neuron Elements/Simple Membrane  ACm=1e-9  ARm=1e7  ECm=1e-9  ERm=1e7  ARFm=1e8  ERFm=1e8
  Sum7 : Sum  SaturateOnIntegerOverflow=on  InputSameDT=on  OutDataTypeStr=Inherit: Same as first input
  Synapse : Subsystem  AncestorBlock=NeuroModelerLibrary/Neuron Elements/Synapse  mask{SecretionTC=0.001, DecompositionTC=0.01, ksi=0.5, gamma=1e8}
      mask prompts: SecretionTC "Mediator Secretion"; DecompositionTC "Mediator Decomposition"
  Synapse1 : Subsystem  AncestorBlock=NeuroModelerLibrary/Neuron Elements/Synapse  mask{SecretionTC=0.001, DecompositionTC=0.01, ksi=0.5, gamma=1e8}
      mask prompts: SecretionTC "Mediator Secretion"; DecompositionTC "Mediator Decomposition"
  Out : Outport
  Visual : Outport  Port=2
  Potential : Outport  Port=3
  wires:
  Synapse1/1(Out1) -> Simple Membrane/5
  Synapse/1(Out1) -> Simple Membrane/1
  Simple Membrane/2 -> Sum7/2
  Simple Membrane/1 -> Sum7/1
  C3/1 -> Simple Membrane/4
  C2/1 -> Simple Membrane/2
  LTZone/1 -> Simple Membrane/3
  Sum7/1 -> Potential/1, LTZone/1
  Arresting/1 -> Synapse1/1(In1)
  Stimulate/1 -> Synapse/1(In1)
  C1/1 -> LTZone/2
  LTZone/3 -> Out/1
  LTZone/2 -> Visual/1

== system RCN_comparation/Pulse Neurons/Subsystem/Simple Cell/Synapse ==
  In1 : Inport
  Constant1 : Constant  Value=0
  Constant4 : Constant  Value=DecompositionTC
  Constant5 : Constant  Value=SecretionTC
  Fcn : Fcn  Expr=u*u*ksi
  Gain : Gain  Gain=4*ksi/gamma  SaturateOnIntegerOverflow=on  OutDataTypeStr=Inherit: Same as input  ParamDataTypeStr=Inherit: Same as input
  Gain1 : Gain  SaturateOnIntegerOverflow=on  OutDataTypeStr=Inherit: Same as input  ParamDataTypeStr=Inherit: Same as input
  Inertial Link : NeuroModelerLibrary/Support/Inertial Link
  Sum : Sum  Inputs=+-  SaturateOnIntegerOverflow=on
  Switch1 : Switch
  Switch2 : Switch  Threshold=1
  Out1 : Outport
  wires:
  Fcn/1 -> Sum/2
  In1/1 -> Switch2/2, Gain1/1
  Sum/1 -> Gain/1
  Inertial Link/1 -> Sum/1
  Constant4/1 -> Switch2/3
  Constant5/1 -> Switch2/1
  Switch2/1 -> Inertial Link/2
  Gain/1 -> Switch1/2, Switch1/1
  Constant1/1 -> Switch1/3
  Gain1/1 -> Inertial Link/1
  Switch1/1 -> Out1/1

== system RCN_comparation/Pulse Neurons/Subsystem/Simple Cell/Synapse1 ==
  In1 : Inport
  Constant1 : Constant  Value=0
  Constant4 : Constant  Value=DecompositionTC
  Constant5 : Constant  Value=SecretionTC
  Fcn : Fcn  Expr=u*u*ksi
  Gain : Gain  Gain=4*ksi/gamma  SaturateOnIntegerOverflow=on  OutDataTypeStr=Inherit: Same as input  ParamDataTypeStr=Inherit: Same as input
  Gain1 : Gain  SaturateOnIntegerOverflow=on  OutDataTypeStr=Inherit: Same as input  ParamDataTypeStr=Inherit: Same as input
  Inertial Link : NeuroModelerLibrary/Support/Inertial Link
  Sum : Sum  Inputs=+-  SaturateOnIntegerOverflow=on
  Switch1 : Switch
  Switch2 : Switch  Threshold=1
  Out1 : Outport
  wires:
  Switch1/1 -> Out1/1
  Gain1/1 -> Inertial Link/1
  Constant1/1 -> Switch1/3
  Gain/1 -> Switch1/1, Switch1/2
  Switch2/1 -> Inertial Link/2
  Constant5/1 -> Switch2/1
  Constant4/1 -> Switch2/3
  Inertial Link/1 -> Sum/1
  Sum/1 -> Gain/1
  In1/1 -> Gain1/1, Switch2/2
  Fcn/1 -> Sum/2

== system RCN_comparation/Pulse Neurons/Subsystem/Simple Cell1/Synapse ==
  In1 : Inport
  Constant1 : Constant  Value=0
  Constant4 : Constant  Value=DecompositionTC
  Constant5 : Constant  Value=SecretionTC
  Fcn : Fcn  Expr=u*u*ksi
  Gain : Gain  Gain=4*ksi/gamma  SaturateOnIntegerOverflow=on  OutDataTypeStr=Inherit: Same as input  ParamDataTypeStr=Inherit: Same as input
  Gain1 : Gain  SaturateOnIntegerOverflow=on  OutDataTypeStr=Inherit: Same as input  ParamDataTypeStr=Inherit: Same as input
  Inertial Link : NeuroModelerLibrary/Support/Inertial Link
  Sum : Sum  Inputs=+-  SaturateOnIntegerOverflow=on
  Switch1 : Switch
  Switch2 : Switch  Threshold=1
  Out1 : Outport
  wires:
  Switch1/1 -> Out1/1
  Gain1/1 -> Inertial Link/1
  Constant1/1 -> Switch1/3
  Gain/1 -> Switch1/1, Switch1/2
  Switch2/1 -> Inertial Link/2
  Constant5/1 -> Switch2/1
  Constant4/1 -> Switch2/3
  Inertial Link/1 -> Sum/1
  Sum/1 -> Gain/1
  In1/1 -> Gain1/1, Switch2/2
  Fcn/1 -> Sum/2

== system RCN_comparation/Pulse Neurons/Subsystem/Simple Cell1/Synapse1 ==
  In1 : Inport
  Constant1 : Constant  Value=0
  Constant4 : Constant  Value=DecompositionTC
  Constant5 : Constant  Value=SecretionTC
  Fcn : Fcn  Expr=u*u*ksi
  Gain : Gain  Gain=4*ksi/gamma  SaturateOnIntegerOverflow=on  OutDataTypeStr=Inherit: Same as input  ParamDataTypeStr=Inherit: Same as input
  Gain1 : Gain  SaturateOnIntegerOverflow=on  OutDataTypeStr=Inherit: Same as input  ParamDataTypeStr=Inherit: Same as input
  Inertial Link : NeuroModelerLibrary/Support/Inertial Link
  Sum : Sum  Inputs=+-  SaturateOnIntegerOverflow=on
  Switch1 : Switch
  Switch2 : Switch  Threshold=1
  Out1 : Outport
  wires:
  Switch1/1 -> Out1/1
  Gain1/1 -> Inertial Link/1
  Constant1/1 -> Switch1/3
  Gain/1 -> Switch1/1, Switch1/2
  Switch2/1 -> Inertial Link/2
  Constant5/1 -> Switch2/1
  Constant4/1 -> Switch2/3
  Inertial Link/1 -> Sum/1
  Sum/1 -> Gain/1
  In1/1 -> Gain1/1, Switch2/2
  Fcn/1 -> Sum/2

== system RCN_comparation/Pulse Neurons/Subsystem/Simple Cell2/Synapse ==
  In1 : Inport
  Constant1 : Constant  Value=0
  Constant4 : Constant  Value=DecompositionTC
  Constant5 : Constant  Value=SecretionTC
  Fcn : Fcn  Expr=u*u*ksi
  Gain : Gain  Gain=4*ksi/gamma  SaturateOnIntegerOverflow=on  OutDataTypeStr=Inherit: Same as input  ParamDataTypeStr=Inherit: Same as input
  Gain1 : Gain  SaturateOnIntegerOverflow=on  OutDataTypeStr=Inherit: Same as input  ParamDataTypeStr=Inherit: Same as input
  Inertial Link : NeuroModelerLibrary/Support/Inertial Link
  Sum : Sum  Inputs=+-  SaturateOnIntegerOverflow=on
  Switch1 : Switch
  Switch2 : Switch  Threshold=1
  Out1 : Outport
  wires:
  Fcn/1 -> Sum/2
  In1/1 -> Switch2/2, Gain1/1
  Sum/1 -> Gain/1
  Inertial Link/1 -> Sum/1
  Constant4/1 -> Switch2/3
  Constant5/1 -> Switch2/1
  Switch2/1 -> Inertial Link/2
  Gain/1 -> Switch1/2, Switch1/1
  Constant1/1 -> Switch1/3
  Gain1/1 -> Inertial Link/1
  Switch1/1 -> Out1/1

== system RCN_comparation/Pulse Neurons/Subsystem/Simple Cell2/Synapse1 ==
  In1 : Inport
  Constant1 : Constant  Value=0
  Constant4 : Constant  Value=DecompositionTC
  Constant5 : Constant  Value=SecretionTC
  Fcn : Fcn  Expr=u*u*ksi
  Gain : Gain  Gain=4*ksi/gamma  SaturateOnIntegerOverflow=on  OutDataTypeStr=Inherit: Same as input  ParamDataTypeStr=Inherit: Same as input
  Gain1 : Gain  SaturateOnIntegerOverflow=on  OutDataTypeStr=Inherit: Same as input  ParamDataTypeStr=Inherit: Same as input
  Inertial Link : NeuroModelerLibrary/Support/Inertial Link
  Sum : Sum  Inputs=+-  SaturateOnIntegerOverflow=on
  Switch1 : Switch
  Switch2 : Switch  Threshold=1
  Out1 : Outport
  wires:
  Switch1/1 -> Out1/1
  Gain1/1 -> Inertial Link/1
  Constant1/1 -> Switch1/3
  Gain/1 -> Switch1/1, Switch1/2
  Switch2/1 -> Inertial Link/2
  Constant5/1 -> Switch2/1
  Constant4/1 -> Switch2/3
  Inertial Link/1 -> Sum/1
  Sum/1 -> Gain/1
  In1/1 -> Gain1/1, Switch2/2
  Fcn/1 -> Sum/2

== system RCN_comparation/Pulse Neurons/Subsystem/Subsystem/"Afferent"1 ==
  Signal : Inport
  Clock : Clock
  Fcn : Fcn  Expr=sin(u)
  Product2 : Product  RndMeth=Zero
  Relay : Relay  OnSwitchValue=0.9  OffSwitchValue=0.9
  Out : Outport
  wires:
  Clock/1 -> Product2/1
  Product2/1 -> Fcn/1
  Signal/1 -> Product2/2
  Fcn/1 -> Relay/1
  Relay/1 -> Out/1

== system RCN_comparation/Pulse Neurons/Subsystem/Subsystem/PAC3 ==
  In1 : Inport
  Constant4 : Constant  Value=DecompositionTC
  Constant5 : Constant  Value=SecretionTC
  Gain1 : Gain  SaturateOnIntegerOverflow=on  OutDataTypeStr=Inherit: Same as input  ParamDataTypeStr=Inherit: Same as input
  Inertial Link : NeuroModelerLibrary/Support/Inertial Link
  Switch2 : Switch  Threshold=1
  Out1 : Outport
  wires:
  In1/1 -> Switch2/2, Gain1/1
  Constant4/1 -> Switch2/3
  Constant5/1 -> Switch2/1
  Switch2/1 -> Inertial Link/2
  Gain1/1 -> Inertial Link/1
  Inertial Link/1 -> Out1/1

== system RCN_comparation/Pulse Neurons/Subsystem/Subsystem/Simple Cell3 ==
  Stimulate : Inport
  Arresting : Inport  Port=2
  C1 : Constant
  C2 : Constant
  C3 : Constant  Value=-1
  LTZone : NeuroModelerLibrary/Neuron Elements/LTZone  NM=1  FB=1.7  IT=0.005  T=0.000001
  Simple Membrane : NeuroModelerLibrary/Neuron Elements/Simple Membrane  ACm=1e-9  ARm=1e7  ECm=1e-9  ERm=1e7  ARFm=1e8  ERFm=1e8
  Sum7 : Sum  SaturateOnIntegerOverflow=on  InputSameDT=on  OutDataTypeStr=Inherit: Same as first input
  Synapse : Subsystem  AncestorBlock=NeuroModelerLibrary/Neuron Elements/Synapse  mask{SecretionTC=0.001, DecompositionTC=0.01, ksi=0.5, gamma=1e8}
      mask prompts: SecretionTC "Mediator Secretion"; DecompositionTC "Mediator Decomposition"
  Synapse1 : Subsystem  AncestorBlock=NeuroModelerLibrary/Neuron Elements/Synapse  mask{SecretionTC=0.001, DecompositionTC=0.01, ksi=0.5, gamma=1e8}
      mask prompts: SecretionTC "Mediator Secretion"; DecompositionTC "Mediator Decomposition"
  Out : Outport
  Visual : Outport  Port=2
  Potential : Outport  Port=3
  wires:
  Synapse1/1(Out1) -> Simple Membrane/5
  Synapse/1(Out1) -> Simple Membrane/1
  Simple Membrane/2 -> Sum7/2
  Simple Membrane/1 -> Sum7/1
  C3/1 -> Simple Membrane/4
  C2/1 -> Simple Membrane/2
  LTZone/1 -> Simple Membrane/3
  Sum7/1 -> Potential/1, LTZone/1
  Arresting/1 -> Synapse1/1(In1)
  Stimulate/1 -> Synapse/1(In1)
  C1/1 -> LTZone/2
  LTZone/3 -> Out/1
  LTZone/2 -> Visual/1

== system RCN_comparation/Pulse Neurons/Subsystem1/Simple Cell3/Synapse ==
  In1 : Inport
  Constant1 : Constant  Value=0
  Constant4 : Constant  Value=DecompositionTC
  Constant5 : Constant  Value=SecretionTC
  Fcn : Fcn  Expr=u*u*ksi
  Gain : Gain  Gain=4*ksi/gamma  SaturateOnIntegerOverflow=on  OutDataTypeStr=Inherit: Same as input  ParamDataTypeStr=Inherit: Same as input
  Gain1 : Gain  SaturateOnIntegerOverflow=on  OutDataTypeStr=Inherit: Same as input  ParamDataTypeStr=Inherit: Same as input
  Inertial Link : NeuroModelerLibrary/Support/Inertial Link
  Sum : Sum  Inputs=+-  SaturateOnIntegerOverflow=on
  Switch1 : Switch
  Switch2 : Switch  Threshold=1
  Out1 : Outport
  wires:
  Fcn/1 -> Sum/2
  In1/1 -> Switch2/2, Gain1/1
  Sum/1 -> Gain/1
  Inertial Link/1 -> Sum/1
  Constant4/1 -> Switch2/3
  Constant5/1 -> Switch2/1
  Switch2/1 -> Inertial Link/2
  Gain/1 -> Switch1/2, Switch1/1
  Constant1/1 -> Switch1/3
  Gain1/1 -> Inertial Link/1
  Switch1/1 -> Out1/1

== system RCN_comparation/Pulse Neurons/Subsystem1/Simple Cell3/Synapse1 ==
  In1 : Inport
  Constant1 : Constant  Value=0
  Constant4 : Constant  Value=DecompositionTC
  Constant5 : Constant  Value=SecretionTC
  Fcn : Fcn  Expr=u*u*ksi
  Gain : Gain  Gain=4*ksi/gamma  SaturateOnIntegerOverflow=on  OutDataTypeStr=Inherit: Same as input  ParamDataTypeStr=Inherit: Same as input
  Gain1 : Gain  SaturateOnIntegerOverflow=on  OutDataTypeStr=Inherit: Same as input  ParamDataTypeStr=Inherit: Same as input
  Inertial Link : NeuroModelerLibrary/Support/Inertial Link
  Sum : Sum  Inputs=+-  SaturateOnIntegerOverflow=on
  Switch1 : Switch
  Switch2 : Switch  Threshold=1
  Out1 : Outport
  wires:
  Switch1/1 -> Out1/1
  Gain1/1 -> Inertial Link/1
  Constant1/1 -> Switch1/3
  Gain/1 -> Switch1/1, Switch1/2
  Switch2/1 -> Inertial Link/2
  Constant5/1 -> Switch2/1
  Constant4/1 -> Switch2/3
  Inertial Link/1 -> Sum/1
  Sum/1 -> Gain/1
  In1/1 -> Gain1/1, Switch2/2
  Fcn/1 -> Sum/2

== system RCN_comparation/Pulse Neurons/Subsystem/Subsystem/Simple Cell3/Synapse ==
  In1 : Inport
  Constant1 : Constant  Value=0
  Constant4 : Constant  Value=DecompositionTC
  Constant5 : Constant  Value=SecretionTC
  Fcn : Fcn  Expr=u*u*ksi
  Gain : Gain  Gain=4*ksi/gamma  SaturateOnIntegerOverflow=on  OutDataTypeStr=Inherit: Same as input  ParamDataTypeStr=Inherit: Same as input
  Gain1 : Gain  SaturateOnIntegerOverflow=on  OutDataTypeStr=Inherit: Same as input  ParamDataTypeStr=Inherit: Same as input
  Inertial Link : NeuroModelerLibrary/Support/Inertial Link
  Sum : Sum  Inputs=+-  SaturateOnIntegerOverflow=on
  Switch1 : Switch
  Switch2 : Switch  Threshold=1
  Out1 : Outport
  wires:
  Fcn/1 -> Sum/2
  In1/1 -> Switch2/2, Gain1/1
  Sum/1 -> Gain/1
  Inertial Link/1 -> Sum/1
  Constant4/1 -> Switch2/3
  Constant5/1 -> Switch2/1
  Switch2/1 -> Inertial Link/2
  Gain/1 -> Switch1/2, Switch1/1
  Constant1/1 -> Switch1/3
  Gain1/1 -> Inertial Link/1
  Switch1/1 -> Out1/1

== system RCN_comparation/Pulse Neurons/Subsystem/Subsystem/Simple Cell3/Synapse1 ==
  In1 : Inport
  Constant1 : Constant  Value=0
  Constant4 : Constant  Value=DecompositionTC
  Constant5 : Constant  Value=SecretionTC
  Fcn : Fcn  Expr=u*u*ksi
  Gain : Gain  Gain=4*ksi/gamma  SaturateOnIntegerOverflow=on  OutDataTypeStr=Inherit: Same as input  ParamDataTypeStr=Inherit: Same as input
  Gain1 : Gain  SaturateOnIntegerOverflow=on  OutDataTypeStr=Inherit: Same as input  ParamDataTypeStr=Inherit: Same as input
  Inertial Link : NeuroModelerLibrary/Support/Inertial Link
  Sum : Sum  Inputs=+-  SaturateOnIntegerOverflow=on
  Switch1 : Switch
  Switch2 : Switch  Threshold=1
  Out1 : Outport
  wires:
  Switch1/1 -> Out1/1
  Gain1/1 -> Inertial Link/1
  Constant1/1 -> Switch1/3
  Gain/1 -> Switch1/1, Switch1/2
  Switch2/1 -> Inertial Link/2
  Constant5/1 -> Switch2/1
  Constant4/1 -> Switch2/3
  Inertial Link/1 -> Sum/1
  Sum/1 -> Gain/1
  In1/1 -> Gain1/1, Switch2/2
  Fcn/1 -> Sum/2
